simulink model "lab2end"  (R2021a)
settings: Solver=VariableStepAuto  StartTime=0.0  StopTime=500  RelTol=1e-3
settings Model: Creator=hamadov  LastModifiedBy=hamadov

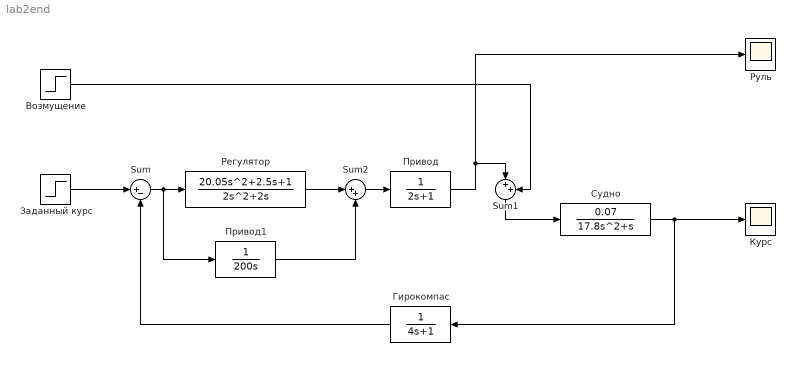
== system lab2end ==
  Sum : Sum  Inputs=|+-
  Sum1 : Sum  Inputs=|++
  Sum2 : Sum  Inputs=|++
  Возмущение : Step  Time=0  After=2  SampleTime=0
  Гирокомпас : TransferFcn  Denominator=[4 1]
  Заданный курс : Step  Time=0  After=10  SampleTime=0
  Курс : Scope
  Привод : TransferFcn  Denominator=[2 1]
  Привод1 : TransferFcn  Denominator=[200 0]
  Регулятор : TransferFcn  Numerator=[20.05 2.5 1]  Denominator=[2 2 0]
  Руль : Scope
  Судно : TransferFcn  Numerator=[0.07]  Denominator=[17.8 1 0]
  wires:
  Привод/1 -> Sum1/1, Руль/1
  Судно/1 -> Курс/1, Гирокомпас/1
  Гирокомпас/1 -> Sum/2
  Sum/1 -> Привод1/1, Регулятор/1
  Заданный курс/1 -> Sum/1
  Sum1/1 -> Судно/1
  Возмущение/1 -> Sum1/2
  Sum2/1 -> Привод/1
  Привод1/1 -> Sum2/2
  Регулятор/1 -> Sum2/1
